simulink model "ART25_old"  (R2022a)
settings: Solver=FixedStepAuto  StartTime=0.0  StopTime=10.0  FixedStep=sim_TimeStep  RelTol=1e-3
undefined symbols (not defined in the file): DiscIntNeverNeededParam, param, param_vdc
libraries: simulink x11
settings Model: Creator=jutri  LastModifiedBy=Usuario
settings ModelReferenceCC: EnableRefExpFcnMdlSchedulingChecks=off
settings RTWCC: Description=Generic Real-Time Target  GPUComputeCapability=5.0

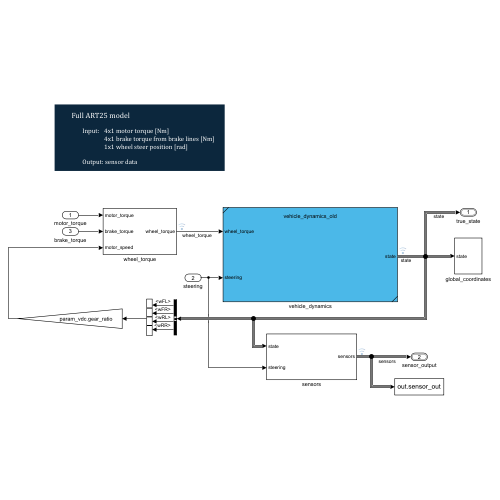
[thumbnail: Simulink's stored preview of the top-level diagram]
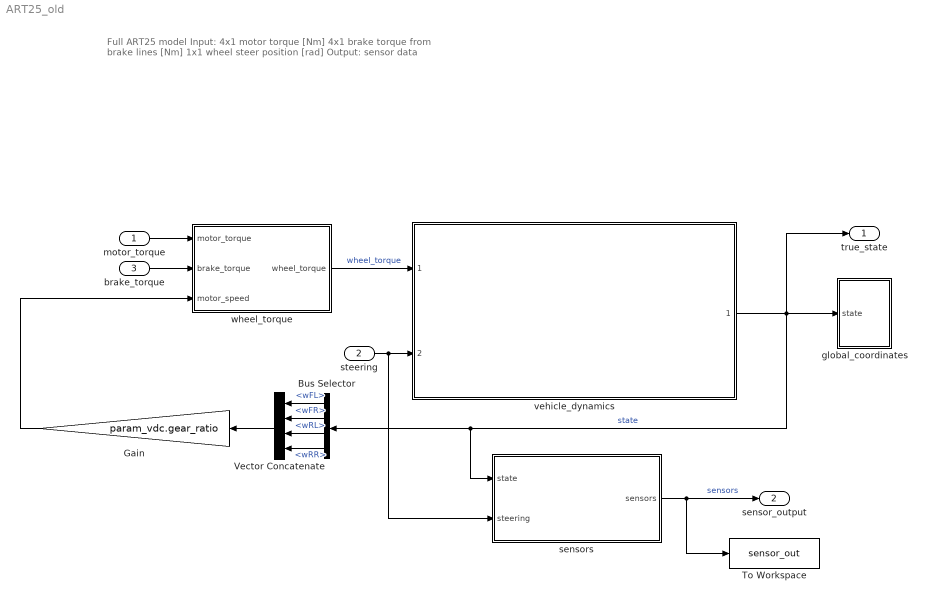
== system ART25_old ==
  note: Full ART25 model
      |
      | Input: 4x1 motor torque [Nm]
      | 4x1 brake torque from brake lines [Nm]
      | 1x1 wheel steer position [rad]
      |
      | Output: sensor data
  motor_torque : Inport  OutDataTypeStr=double  PortDimensions=[4,1]
  steering : Inport  Port=2
  brake_torque : Inport  Port=3  OutDataTypeStr=double  PortDimensions=[4,1]
  Bus Selector : BusSelector  OutputSignals=wFL,wFR,wRL,wRR
  Gain : Gain  Gain=param_vdc.gear_ratio
  To Workspace : ToWorkspace  VariableName=sensor_out  SaveFormat=Timeseries  SampleTime=-1
  Vector Concatenate : Concatenate  NumInputs=4
  global_coordinates : Subsystem
  sensors : Subsystem
  vehicle_dynamics : Subsystem  ReferencedSubsystem=vehicle_dynamics_old
  wheel_torque : Subsystem
  true_state : Outport  OutDataTypeStr=Bus: stateBus
  sensor_output : Outport  Port=2  OutDataTypeStr=Bus: sensorBus
  wires:
  sensors/1(sensors) -> To Workspace/1, sensor_output/1  "sensors"
  wheel_torque/1(wheel_torque) -> vehicle_dynamics/1  "wheel_torque"
  steering/1 -> sensors/2(steering), vehicle_dynamics/2
  motor_torque/1 -> wheel_torque/1(motor_torque)
  brake_torque/1 -> wheel_torque/2(brake_torque)
  vehicle_dynamics/1 -> sensors/1(state), Bus Selector/1, true_state/1, global_coordinates/1(state)  "state"
  Bus Selector/1 -> Vector Concatenate/1  "<wFL>"
  Bus Selector/2 -> Vector Concatenate/2  "<wFR>"
  Bus Selector/3 -> Vector Concatenate/3  "<wRL>"
  Bus Selector/4 -> Vector Concatenate/4  "<wRR>"
  Vector Concatenate/1 -> Gain/1
  Gain/1 -> wheel_torque/3(motor_speed)

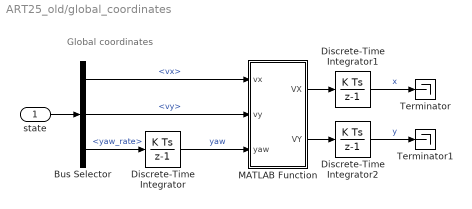
== system ART25_old/global_coordinates ==
  note: Global coordinates
  state : Inport
  Bus Selector : BusSelector  OutputSignals=vx,vy,yaw_rate
  Discrete-Time Integrator : DiscreteIntegrator  SampleTime=-1  ICPrevOutput=DiscIntNeverNeededParam  ICPrevScaledInput=DiscIntNeverNeededParam
  Discrete-Time Integrator1 : DiscreteIntegrator  SampleTime=-1  ICPrevOutput=DiscIntNeverNeededParam  ICPrevScaledInput=DiscIntNeverNeededParam
  Discrete-Time Integrator2 : DiscreteIntegrator  SampleTime=-1  ICPrevOutput=DiscIntNeverNeededParam  ICPrevScaledInput=DiscIntNeverNeededParam
  MATLAB Function : MATLAB Function  TreatAsAtomicUnit=on
  Terminator : Terminator
  Terminator1 : Terminator
  wires:
  Bus Selector/2 -> MATLAB Function/2(vy)  "<vy>"
  Bus Selector/3 -> Discrete-Time Integrator/1  "<yaw_rate>"
  Discrete-Time Integrator/1 -> MATLAB Function/3(yaw)  "yaw"
  MATLAB Function/2(VY) -> Discrete-Time Integrator2/1
  Discrete-Time Integrator1/1 -> Terminator/1  "x"
  Discrete-Time Integrator2/1 -> Terminator1/1  "y"
  MATLAB Function/1(VX) -> Discrete-Time Integrator1/1
  Bus Selector/1 -> MATLAB Function/1(vx)  "<vx>"
  state/1 -> Bus Selector/1

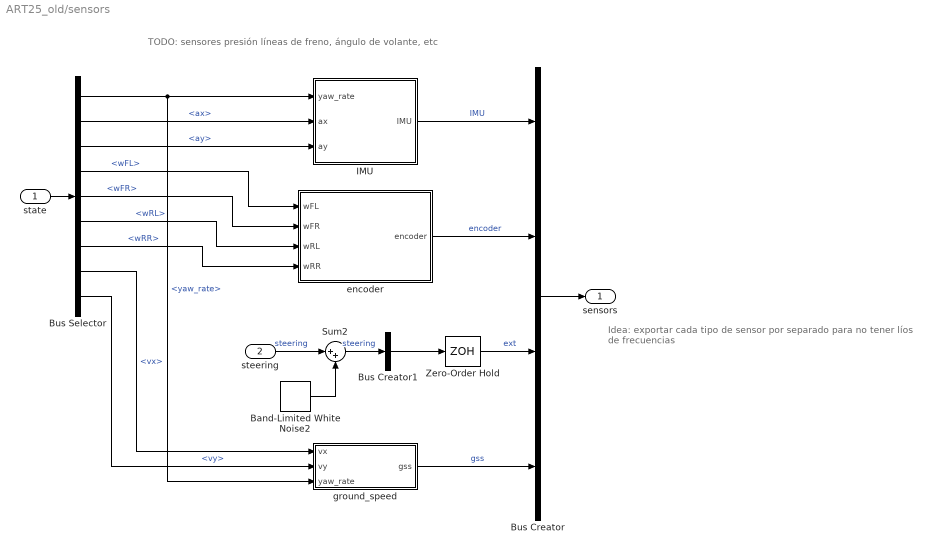
== system ART25_old/sensors ==
  note: Idea: exportar cada tipo de sensor por separado para no tener
      | líos de frecuencias
  note: TODO: sensores presión líneas de freno, ángulo de volante, etc
  state : Inport
  steering : Inport  Port=2
  Band-Limited White Noise2 : simulink/Sources/Band-Limited White Noise  Cov=param.sensors.ext_sigma^2  Ts=param.sensors.ext_hz  seed=[23341]
  Bus Creator : BusCreator  Inputs=4
  Bus Creator1 : BusCreator  Inputs=1
  Bus Selector : BusSelector  OutputSignals=yaw_rate,ax,ay,wFL,wFR,wRL,wRR,vx,vy
  IMU : Subsystem
  Sum2 : Sum  Inputs=|++
  Zero-Order Hold : ZeroOrderHold  SampleTime=param.sensors.ext_hz
  encoder : Subsystem
  ground_speed : Subsystem
  sensors : Outport
  wires:
  state/1 -> Bus Selector/1
  Bus Selector/4 -> encoder/1(wFL)  "<wFL>"
  Bus Selector/5 -> encoder/2(wFR)  "<wFR>"
  Bus Selector/6 -> encoder/3(wRL)  "<wRL>"
  Bus Selector/7 -> encoder/4(wRR)  "<wRR>"
  Bus Selector/1 -> ground_speed/3(yaw_rate), IMU/1(yaw_rate)  "<yaw_rate>"
  Bus Selector/2 -> IMU/2(ax)  "<ax>"
  Bus Selector/3 -> IMU/3(ay)  "<ay>"
  Bus Creator/1 -> sensors/1
  IMU/1(IMU) -> Bus Creator/1  "IMU"
  encoder/1(encoder) -> Bus Creator/2  "encoder"
  Sum2/1 -> Bus Creator1/1  "steering"
  Bus Creator1/1 -> Zero-Order Hold/1
  Band-Limited White Noise2/1 -> Sum2/2
  steering/1 -> Sum2/1  "steering"
  Zero-Order Hold/1 -> Bus Creator/3  "ext"
  ground_speed/1(gss) -> Bus Creator/4  "gss"
  Bus Selector/8 -> ground_speed/1(vx)  "<vx>"
  Bus Selector/9 -> ground_speed/2(vy)  "<vy>"

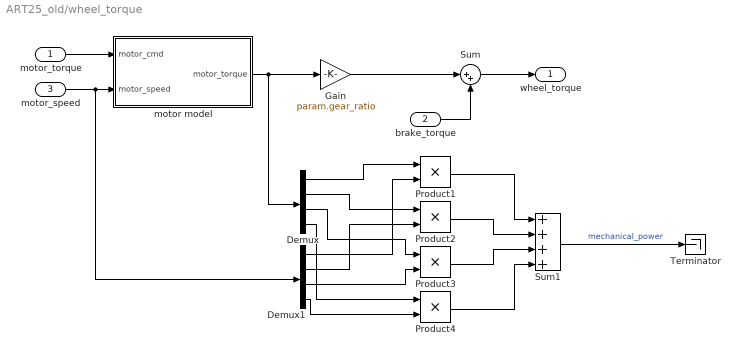
== system ART25_old/wheel_torque ==
  motor_torque : Inport
  brake_torque : Inport  Port=2
  motor_speed : Inport  Port=3
  Demux : Demux
  Demux1 : Demux
  Gain : Gain  Gain=param.gear_ratio
  Product{1..4} (4 alike) : Product
  Sum : Sum  Inputs=|++
  Sum1 : Sum  Inputs=++++
  Terminator : Terminator
  motor model : Subsystem
  wheel_torque : Outport
  wires:
  Sum/1 -> wheel_torque/1
  brake_torque/1 -> Sum/2
  motor_torque/1 -> motor model/1(motor_cmd)
  Gain/1 -> Sum/1
  motor model/1(motor_torque) -> Demux/1, Gain/1
  motor_speed/1 -> Demux1/1, motor model/2(motor_speed)
  Sum1/1 -> Terminator/1  "mechanical_power"
  Demux/1 -> Product1/1
  Demux1/1 -> Product1/2
  Demux/2 -> Product2/1
  Demux1/2 -> Product2/2
  Demux/3 -> Product3/1
  Demux1/3 -> Product3/2
  Demux/4 -> Product4/1
  Demux1/4 -> Product4/2
  Product2/1 -> Sum1/2
  Product3/1 -> Sum1/3
  Product4/1 -> Sum1/4
  Product1/1 -> Sum1/1

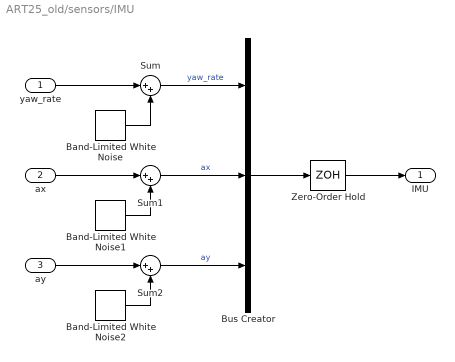
== system ART25_old/sensors/IMU ==
  yaw_rate : Inport
  ax : Inport  Port=2
  ay : Inport  Port=3
  Band-Limited White Noise : simulink/Sources/Band-Limited White Noise  Cov=param.sensors.IMU_sigma_gyro^2  Ts=param.sensors.IMU_hz  seed=[23331]
  Band-Limited White Noise1 : simulink/Sources/Band-Limited White Noise  Cov=param.sensors.IMU_sigma_accel^2  Ts=param.sensors.IMU_hz  seed=[23342]
  Band-Limited White Noise2 : simulink/Sources/Band-Limited White Noise  Cov=param.sensors.IMU_sigma_accel^2  Ts=param.sensors.IMU_hz  seed=[23341]
  Bus Creator : BusCreator  Inputs=3
  Sum : Sum  Inputs=|++
  Sum1 : Sum  Inputs=|++
  Sum2 : Sum  Inputs=|++
  Zero-Order Hold : ZeroOrderHold  SampleTime=param.sensors.IMU_hz
  IMU : Outport
  wires:
  yaw_rate/1 -> Sum/1
  Band-Limited White Noise/1 -> Sum/2
  Sum/1 -> Bus Creator/1  "yaw_rate"
  Bus Creator/1 -> Zero-Order Hold/1
  Sum1/1 -> Bus Creator/2  "ax"
  Band-Limited White Noise1/1 -> Sum1/2
  ax/1 -> Sum1/1
  ay/1 -> Sum2/1
  Band-Limited White Noise2/1 -> Sum2/2
  Sum2/1 -> Bus Creator/3  "ay"
  Zero-Order Hold/1 -> IMU/1

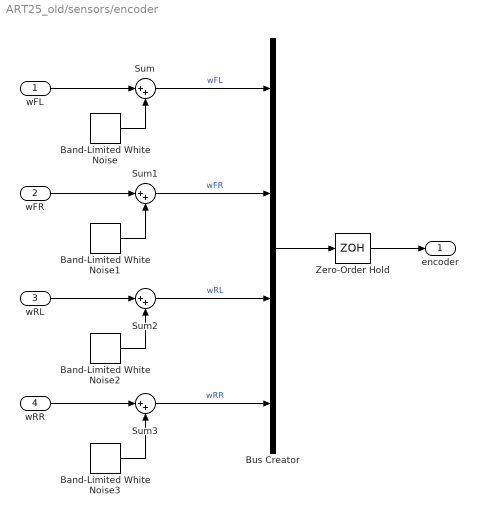
== system ART25_old/sensors/encoder ==
  wFL : Inport
  wFR : Inport  Port=2
  wRL : Inport  Port=3
  wRR : Inport  Port=4
  Band-Limited White Noise{,1..3} (4 alike) : simulink/Sources/Band-Limited White Noise  Cov=param.sensors.encoder_sigma^2  Ts=param.sensors.encoder_hz  seed=[23341]
  Bus Creator : BusCreator  Inputs=4
  Sum{,1..3} (4 alike) : Sum  Inputs=|++
  Zero-Order Hold : ZeroOrderHold  SampleTime=param.sensors.encoder_hz
  encoder : Outport
  wires:
  wFL/1 -> Sum/1
  Band-Limited White Noise/1 -> Sum/2
  Sum/1 -> Bus Creator/1  "wFL"
  Sum1/1 -> Bus Creator/2  "wFR"
  Band-Limited White Noise1/1 -> Sum1/2
  wFR/1 -> Sum1/1
  wRL/1 -> Sum2/1
  Band-Limited White Noise2/1 -> Sum2/2
  Sum2/1 -> Bus Creator/3  "wRL"
  Sum3/1 -> Bus Creator/4  "wRR"
  Band-Limited White Noise3/1 -> Sum3/2
  wRR/1 -> Sum3/1
  Bus Creator/1 -> Zero-Order Hold/1
  Zero-Order Hold/1 -> encoder/1

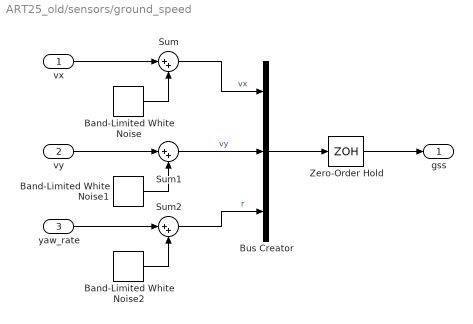
== system ART25_old/sensors/ground_speed ==
  vx : Inport
  vy : Inport  Port=2
  yaw_rate : Inport  Port=3
  Band-Limited White Noise : simulink/Sources/Band-Limited White Noise  Cov=param.sensors.gss_sigma^2  Ts=param.sensors.gss_hz  seed=[23341]
  Band-Limited White Noise1 : simulink/Sources/Band-Limited White Noise  Cov=(param.sensors.gss_sigma*0.8/20)^2  Ts=param.sensors.gss_hz  seed=[23342]
  Band-Limited White Noise2 : simulink/Sources/Band-Limited White Noise  Cov=(param.sensors.gss_sigma*0.8/20)^2  Ts=param.sensors.gss_hz  seed=[23343]
  Bus Creator : BusCreator  Inputs=3
  Sum : Sum  Inputs=|++
  Sum1 : Sum  Inputs=|++
  Sum2 : Sum  Inputs=|++
  Zero-Order Hold : ZeroOrderHold  SampleTime=param.sensors.gss_hz
  gss : Outport
  wires:
  Band-Limited White Noise1/1 -> Sum1/2
  vx/1 -> Sum/1
  Zero-Order Hold/1 -> gss/1
  Bus Creator/1 -> Zero-Order Hold/1
  Sum1/1 -> Bus Creator/2  "vy"
  Band-Limited White Noise/1 -> Sum/2
  Sum/1 -> Bus Creator/1  "vx"
  vy/1 -> Sum1/1
  yaw_rate/1 -> Sum2/1
  Band-Limited White Noise2/1 -> Sum2/2
  Sum2/1 -> Bus Creator/3  "r"

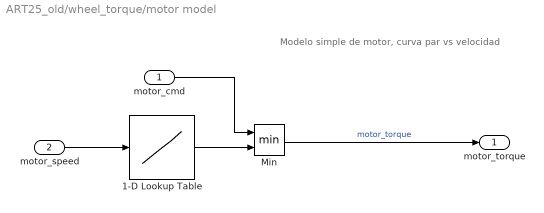
== system ART25_old/wheel_torque/motor model ==
  note: Modelo simple de motor, curva par vs velocidad
  motor_cmd : Inport
  motor_speed : Inport  Port=2
  1-D Lookup Table : Lookup_n-D  NumberOfTableDimensions=1  BreakpointsForDimension1=[0 16000 19900 20000]*pi/30  Table=[21 21 13 0]  InternalRulePriority=Speed  RndMeth=Simplest
  Min : MinMax  Inputs=2
  motor_torque : Outport
  wires:
  motor_cmd/1 -> Min/1
  motor_speed/1 -> 1-D Lookup Table/1
  1-D Lookup Table/1 -> Min/2
  Min/1 -> motor_torque/1  "motor_torque"

== matlab function ART25_old/global_coordinates/MATLAB Function ==
  data: vx input; vy input; yaw input; VX output; VY output
function [VX, VY] = fcn(vx, vy, yaw)

VX = vx*cos(yaw) - vy*sin(yaw);
VY = vx*sin(yaw) + vy*cos(yaw);
